simulink library "csu_tfm_tether_mtv"  (R2014b)
settings: Solver=ode45  StartTime=0.0  StopTime=10.0  RelTol=1e-3
values from neighbouring files (symbols this model uses):
  tfm_attachment_location_body = [0.0 0.0 0.2]    [csu_tfm_tether_model_init.m]
  tfm_cg_enable = 1    [csu_tfm_tether_model_init.m]
  tfm_forces_enable = 1    [csu_tfm_tether_model_init.m]
  tfm_hanging_location_topo = [0.0 0.0 10.0]    [csu_tfm_tether_model_init.m]
  tfm_horseshoe_bolt_mass = 0.5    [csu_tfm_tether_model_init.m]
  tfm_moments_enable = 1    [csu_tfm_tether_model_init.m]
  tfm_sleeve_mass = 0.5    [csu_tfm_tether_model_init.m]
  tfm_tether_mass_per_length = 1.0    (= 1)    [csu_tfm_tether_model_init.m]
  tfm_tether_spring_constant = 10.0    (= 10)    [csu_tfm_tether_model_init.m]
  tfm_tether_unstretched_length = 9.21    [csu_tfm_tether_model_init.m]
libraries: simulink x2, util_common_lib x2, util_quat_lib x2
settings Model: Creator=Mark Wells  LastModifiedBy=Mark Wells

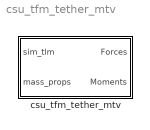
== system csu_tfm_tether_mtv ==
  csu_tfm_tether_mtv : Subsystem

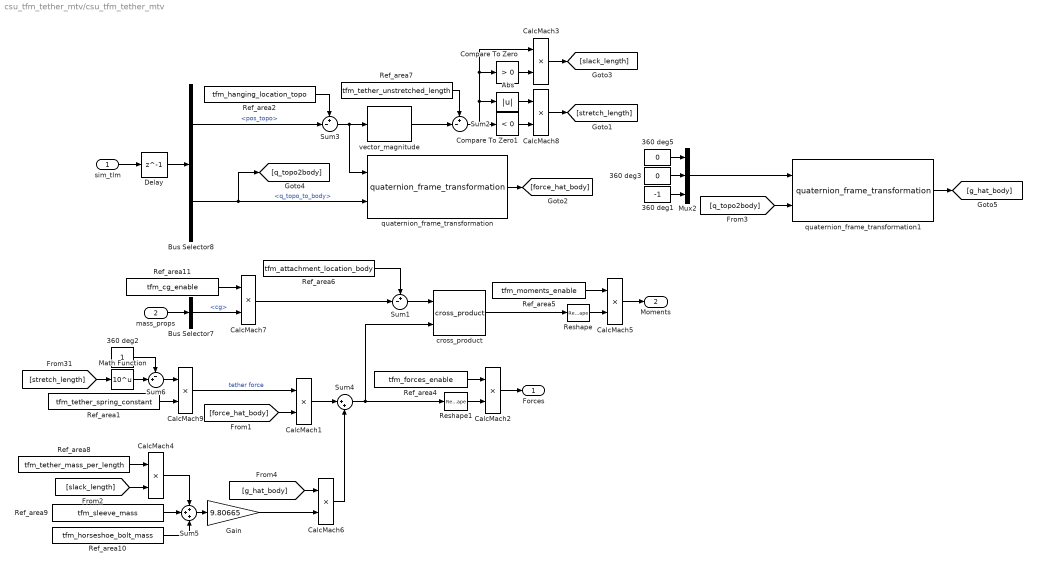
== system csu_tfm_tether_mtv/csu_tfm_tether_mtv ==
  sim_tlm : Inport
  mass_props : Inport  Port=2
  360 deg1 : Constant  Value=-1
  360 deg2 : Constant
  360 deg3 : Constant  Value=0
  360 deg5 : Constant  Value=0
  Abs : Abs
  Bus Selector7 : BusSelector  OutputSignals=cg
  Bus Selector8 : BusSelector  OutputSignals=pos_topo,q_topo_to_body
  CalcMach{1..9} (9 alike) : Product  SaturateOnIntegerOverflow=on  OutDataTypeStr=Inherit: Same as first input
  Compare To Zero : simulink/Logic and Bit Operations/Compare To Zero  relop=>  OutDataTypeStr=uint8
  Compare To Zero1 : simulink/Logic and Bit Operations/Compare To Zero  relop=<  OutDataTypeStr=uint8
  Delay : Delay  DelayLength=1
  Gain : Gain  Gain=9.80665
  Math Function : Math  Operator=10^u  SaturateOnIntegerOverflow=on
  Mux2 : Mux  Inputs=3
  Ref_area1 : Constant  Value=tfm_tether_spring_constant
  Ref_area10 : Constant  Value=tfm_horseshoe_bolt_mass
  Ref_area11 : Constant  Value=tfm_cg_enable
  Ref_area2 : Constant  Value=tfm_hanging_location_topo
  Ref_area4 : Constant  Value=tfm_forces_enable
  Ref_area5 : Constant  Value=tfm_moments_enable
  Ref_area6 : Constant  Value=tfm_attachment_location_body
  Ref_area7 : Constant  Value=tfm_tether_unstretched_length
  Ref_area8 : Constant  Value=tfm_tether_mass_per_length
  Ref_area9 : Constant  Value=tfm_sleeve_mass
  Reshape : Reshape
  Reshape1 : Reshape
  Sum1 : Sum  Inputs=+-|
  Sum2 : Sum  Inputs=+-|
  Sum3 : Sum  Inputs=+-|
  Sum4 : Sum  Inputs=|++
  Sum5 : Sum  Inputs=+++
  Sum6 : Sum  Inputs=-+|
  cross_product : util_common_lib/cross_product  SystemSampleTime=-1
  quaternion_frame_transformation : util_quat_lib/quaternion_frame_transformation  SystemSampleTime=-1
  quaternion_frame_transformation1 : util_quat_lib/quaternion_frame_transformation  SystemSampleTime=-1
  vector_magnitude : util_common_lib/vector_magnitude  SystemSampleTime=-1
  Forces : Outport
  Moments : Outport  Port=2
  wires:
  360 deg2/1 -> Sum6/1
  Sum6/1 -> CalcMach9/1
  CalcMach6/1 -> Sum4/2
  CalcMach1/1 -> Sum4/1
  Abs/1 -> CalcMach8/1
  Compare To Zero1/1 -> CalcMach8/2
  Compare To Zero/1 -> CalcMach3/2
  CalcMach8/1 -> [stretch_length]
  Math Function/1 -> Sum6/2
  CalcMach7/1 -> Sum1/2
  Bus Selector7/1 -> CalcMach7/2  "<cg>"
  Ref_area11/1 -> CalcMach7/1
  Delay/1 -> Bus Selector8/1
  sim_tlm/1 -> Delay/1
  Reshape1/1 -> CalcMach2/2
  Reshape/1 -> CalcMach5/2
  Sum5/1 -> Gain/1
  Ref_area10/1 -> Sum5/3
  CalcMach4/1 -> Sum5/1
  Ref_area9/1 -> Sum5/2
  Sum4/1 -> cross_product/2, Reshape1/1
  [slack_length] -> CalcMach4/2
  [g_hat_body] -> CalcMach6/1
  quaternion_frame_transformation1/1 -> [g_hat_body]
  360 deg1/1 -> Mux2/3
  Ref_area8/1 -> CalcMach4/1
  [q_topo2body] -> quaternion_frame_transformation1/2
  360 deg5/1 -> Mux2/1
  360 deg3/1 -> Mux2/2
  Mux2/1 -> quaternion_frame_transformation1/1
  mass_props/1 -> Bus Selector7/1
  Bus Selector8/1 -> Sum3/2  "<pos_topo>"
  vector_magnitude/1 -> Sum2/2
  Ref_area2/1 -> Sum3/1
  [stretch_length] -> Math Function/1
  Ref_area1/1 -> CalcMach9/2
  Bus Selector8/2 -> [q_topo2body], quaternion_frame_transformation/2  "<q_topo_to_body>"
  quaternion_frame_transformation/1 -> [force_hat_body]
  Ref_area4/1 -> CalcMach2/1
  CalcMach2/1 -> Forces/1
  [force_hat_body] -> CalcMach1/2
  CalcMach9/1 -> CalcMach1/1  "tether force"
  CalcMach5/1 -> Moments/1
  Ref_area6/1 -> Sum1/1
  Sum1/1 -> cross_product/1
  Ref_area5/1 -> CalcMach5/1
  cross_product/1 -> Reshape/1
  Ref_area7/1 -> Sum2/1
  Sum2/1 -> Compare To Zero1/1, Abs/1, Compare To Zero/1, CalcMach3/1
  CalcMach3/1 -> [slack_length]
  Sum3/1 -> quaternion_frame_transformation/1, vector_magnitude/1
  Gain/1 -> CalcMach6/2
